simulink model "PID_task3"  (R2020b)
settings: Solver=VariableStepAuto  StartTime=0.0  StopTime=3  RelTol=1e-3
values from neighbouring files (symbols this model uses):
  den = (mp*s^2+(cp+cs)*s+(kp+ks))*(ms*s^2+cs*s+ks)-(cs*s+ks)^2    [Copy_of_Lab_3_ale.m]    (also in Lab_3_ale.m; mass_2dof.m)
  hd = 1.5    [Copy_of_Lab_3_ale.m]    (also in Lab_3_ale.m)
  hi = 0    [Copy_of_Lab_3_ale.m]    (also in Lab_3_ale.m = 0.2)
  hp = 0    [Copy_of_Lab_3_ale.m]    (also in Lab_3_ale.m)
  kp = 6.32    [Copy_of_Lab_3_ale.m]    (also in Lab_3_ale.m; mass_2dof.m)
  mp = 0.16    [Copy_of_Lab_3_ale.m]    (also in Lab_3_ale.m; mass_2dof.m)
  num = (s*cp+kp)*(s*cs+ks)    [Copy_of_Lab_3_ale.m]    (also in Lab_3_ale.m; mass_2dof.m)
  wn = wn_und_1dof    [Copy_of_Lab_3_ale.m]    (also in H_inf_ctrl_11_2.m = eig(Ask); H_inf_ctrl_11_2_m.m = eig(Ask); Lab_3_ale.m = sqrt(kp/mp); mass_2dof.m)
undefined symbols (not defined in the file or in its folder): sigbuilder_block
settings Model: Creator=tawsi_000  LastModifiedBy=tawsi_000
settings DebuggingCC: UnconnectedInputMsg=none  UnconnectedOutputMsg=none  UnconnectedLineMsg=none  SFMachineParentedDataDiag=error
settings ModelReferenceCC: EnableRefExpFcnMdlSchedulingChecks=off

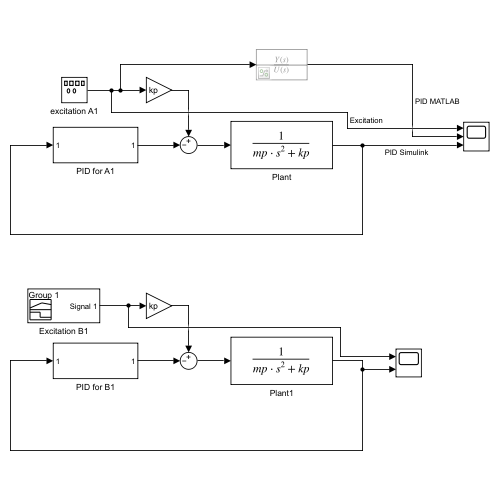
[thumbnail: Simulink's stored preview of the top-level diagram]
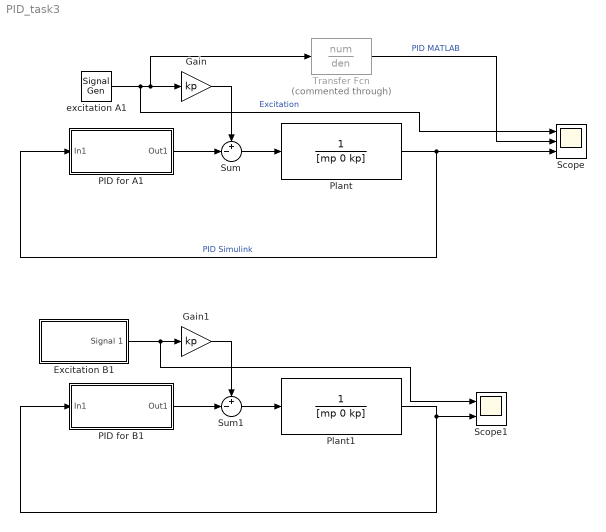
== system PID_task3 ==
  Excitation B1 : Subsystem  Tag=STV Subsys  LoadFcn=sigbuilder_block('load');  StartFcn=sigbuilder_block('start');  StopFcn=sigbuilder_block('stop');  ClipboardFcn=sigbuilder_block('clipboard');  mask(Sigbuilder block){tuvar=[0:10]}
      mask help: Simulink:masks:SigbuilderBlock_MD
      mask init:
      | if ~strcmp(get_param(bdroot(gcbh),'SimulationStatus'),'stopped') tuvar = sigbuilder_block('maskInit'); end
      settings: CopyFcn=sigbuilder_block('copy');  DeleteFcn=sigbuilder_block('delete');  ModelCloseFcn=sigbuilder_block('modelClose');  PreSaveFcn=sigbuilder_block('preSave');  PauseFcn=sigbuilder_block('pause');  ContinueFcn=sigbuilder_block('continue');  NameChangeFcn=sigbuilder_block('namechange');  OpenFcn=sigbuilder_block('open',[437.6 199.2 550.4 400 ]);  CloseFcn=sigbuilder_block('close');
      mask Display: plot(0, 0, 100, 100,[2, 2, 32, 32, 2], [68, 8, 8, 68, 68],[32, 2], [38, 38], [32, 19, 2],[53, 60, 44], [32, 17, 17, 2],[16, 16, 31, 31]);txt = getActiveGroup(gcbh);text(2, 100, txt,'verticalAlignment', 'top');
  Gain : Gain  Gain=kp
  Gain1 : Gain  Gain=kp
  PID for A1 : Subsystem
  PID for B1 : Subsystem
  Plant : TransferFcn  Denominator=[mp 0 kp]
  Plant1 : TransferFcn  Denominator=[mp 0 kp]
  Scope : Scope  NumInputPorts=3
  Scope1 : Scope  NumInputPorts=2
  Sum : Sum  Inputs=+-|
  Sum1 : Sum  Inputs=+-|
  Transfer Fcn : TransferFcn  Commented=through  Numerator=num  Denominator=den
  excitation A1 : SignalGenerator  Amplitude=0.05  Frequency=wn  Units=rad/sec
  wires:
  Plant/1 -> PID for A1/1(In1), Scope/3  "PID Simulink"
  PID for A1/1(Out1) -> Sum/2
  excitation A1/1 -> Scope/1, Transfer Fcn/1, Gain/1  "Excitation"
  Sum/1 -> Plant/1
  Gain/1 -> Sum/1
  Excitation B1/1(Signal 1) -> Scope1/1, Gain1/1
  Sum1/1 -> Plant1/1
  Gain1/1 -> Sum1/1
  PID for B1/1(Out1) -> Sum1/2
  Plant1/1 -> PID for B1/1(In1), Scope1/2
  Transfer Fcn/1 -> Scope/2  "PID MATLAB"

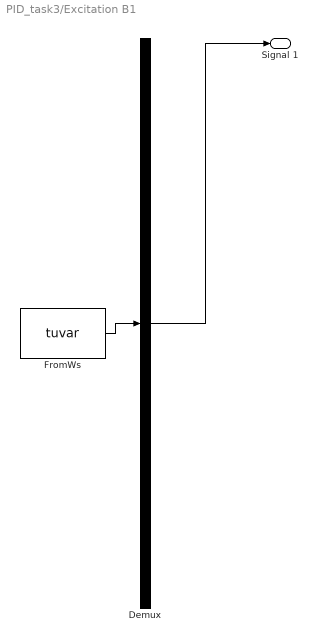
== system PID_task3/Excitation B1 ==
  Demux : Demux  Tag=STV Demux  Outputs=1
      settings: DisplayOption=none
  FromWs : FromWorkspace  Tag=STV FromWs  VariableName=tuvar
      SigBuilderData=|
      | common.afterFinalStr = 'Extrapolate'
      | common.sampleTime = 0
      | dataSet.timeRange = [0 10]
      | dataSet.name = 'Group 1'
      | sbobj.Groups.Name = 'Group 1'
      | sbobj.Groups.Signals.Name = 'Signal 1'
      | sbobj.Groups.Signals.XData = [0 4 4 4.1 4.1 10]
      | sbobj.Groups.Signals.YData = [0 0 0.05 0.05 0 0]
  Signal 1 : Outport  Tag=STV Outport
  wires:
  FromWs/1 -> Demux/1
  Demux/1 -> Signal 1/1

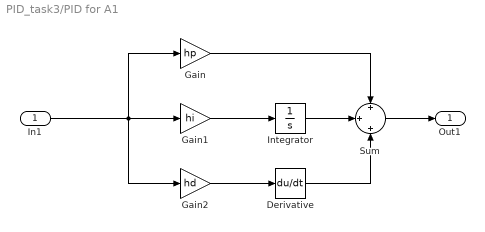
== system PID_task3/PID for A1 ==
  In1 : Inport
  Derivative : Derivative
  Gain : Gain  Gain=hp
  Gain1 : Gain  Gain=hi
  Gain2 : Gain  Gain=hd
  Integrator : Integrator
  Sum : Sum  Inputs=+|+|+
  Out1 : Outport
  wires:
  Sum/1 -> Out1/1
  Gain/1 -> Sum/1
  Gain1/1 -> Integrator/1
  Integrator/1 -> Sum/2
  Gain2/1 -> Derivative/1
  Derivative/1 -> Sum/3
  In1/1 -> Gain2/1, Gain/1, Gain1/1

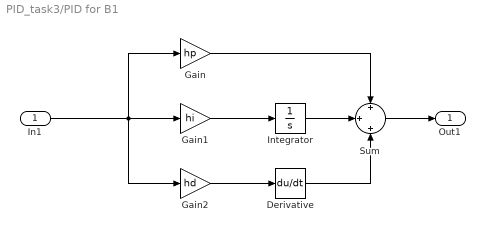
== system PID_task3/PID for B1 ==
  In1 : Inport
  Derivative : Derivative
  Gain : Gain  Gain=hp
  Gain1 : Gain  Gain=hi
  Gain2 : Gain  Gain=hd
  Integrator : Integrator
  Sum : Sum  Inputs=+|+|+
  Out1 : Outport
  wires:
  Sum/1 -> Out1/1
  Gain/1 -> Sum/1
  Gain1/1 -> Integrator/1
  Integrator/1 -> Sum/2
  Gain2/1 -> Derivative/1
  Derivative/1 -> Sum/3
  In1/1 -> Gain2/1, Gain/1, Gain1/1
